simulink library "UserContent_lib"  (Simulink 7.8)
settings: Solver=ode45  SolverMode=SingleTasking  StartTime=0.0  StopTime=10.0  RelTol=1e-3
undefined symbols (not defined in the file): bias, ln, Timestep, u_gain_light, u_gain_moderate, u_gain_severe, v_gain_light, v_gain_moderate, v_gain_severe, w_gain_light, w_gain_moderate, w_gain_severe, WindDir, WindSpd
libraries: simulink x8
(part 2 of 2)

== system UserContent_lib/Input Generator/Winds/Turbulence  Model/Dryden Model/Longitudinal Turbulence/filter parameters/Tm-4511 severe data ==
  note: "Light" and "Moderate" sigmas are ZERO below 1km alt.
      | Table 2-79 does not define them.
  "alt, m" : Inport
  intensity : Inport  Port=2
  "Longitudinal Scale, m TM-4511 Table 2-79" : Lookup  InputValues=[0 10 20 30 40 50 60 70 80 90 100 200 304.8 305 762 769 900 1000 2000 4000 6000 8000 10000 12000 14000 16000]  Table=[21 21 33 43 52 61 68 75 82 89 95 149 196 300 300 533 533 832 902 1040 1040 1040 1230 1800 2820 3400]  SaturateOnIntegerOverflow=on
  "Longitudinal sigma, m/s light TM-4511 Table 2-79" : Lookup  InputValues="[10 20 30 40 50 60 70 80 90 100 200 304.8 305 400  762 769 1000 2000 4000 6000 8000 10000 12000 14000 16000]"  Table="[0   0   0   0   0   0   0   0   0    0    0    0   0   0   0   0   .17  .17  .2   .21   .22   .22   .25   .26   .24   ]"  SaturateOnIntegerOverflow=on
  "Longitudinal sigma, m/s moderate TM-4511 Table 2-79" : Lookup  InputValues="[10 20 30 40 50 60 70 80 90 100 200 304.8 305 400  762 769 1000 2000 4000 6000 8000 10000 12000 14000 16000]"  Table="[0   0  0    0    0   0  0  0   0   0     0    0      0     0      0    0  1.65  1.65 2.04 2.13 2.15 2.23 2.47 2.62 2.44]"  SaturateOnIntegerOverflow=on
  "Longitudinal sigma, m/s severe TM-4511 Table 2-79" : Lookup  InputValues="[10 20 30 40 50 60 70 80 90 100 200 304.8 305 400  762 769 1000 2000 4000 6000 8000 10000 12000 14000 16000]"  Table=[2.31 2.58 2.75 2.88 2.98 3.07 3.15 3.22 3.28 3.33 3.72 3.95 4.37 4.39 4.39 5.7 5.7 5.8 6.24 7.16 7.59 7.72 7.89 6.93 5]  SaturateOnIntegerOverflow=on
  Multiport Switch : MultiPortSwitch  zeroidx=off  SaturateOnIntegerOverflow=on  InputSameDT=on
  "sigma, m/s" : Outport
  "scale length, m" : Outport  Port=2
  wires:
  intensity/1 -> Multiport Switch/1
  "Longitudinal sigma, m/s light TM-4511 Table 2-79"/1 -> Multiport Switch/2
  "Longitudinal sigma, m/s moderate TM-4511 Table 2-79"/1 -> Multiport Switch/3
  "Longitudinal sigma, m/s severe TM-4511 Table 2-79"/1 -> Multiport Switch/4
  Multiport Switch/1 -> "sigma, m/s"/1
  "Longitudinal Scale, m TM-4511 Table 2-79"/1 -> "scale length, m"/1
  "alt, m"/1 -> "Longitudinal sigma, m/s light TM-4511 Table 2-79"/1, "Longitudinal sigma, m/s moderate TM-4511 Table 2-79"/1, "Longitudinal Scale, m TM-4511 Table 2-79"/1, "Longitudinal sigma, m/s severe TM-4511 Table 2-79"/1

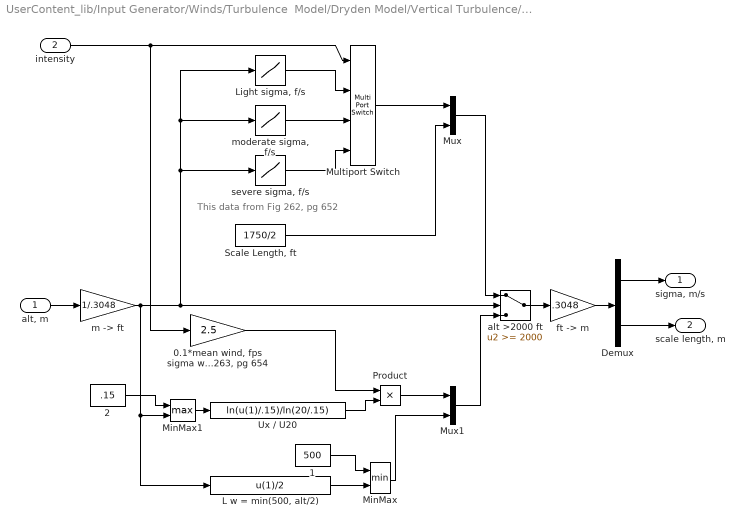
== system UserContent_lib/Input Generator/Winds/Turbulence  Model/Dryden Model/Vertical Turbulence/SubSystem/MIL-STD-1797A APPENDIX A  ==
  note: This data from Fig 262, pg 652
  "alt, m" : Inport
  intensity : Inport  Port=2
  "0.1*mean wind, fps sigma w = to 2.5f/s * intensity Fig 263, pg 654" : Gain  Gain=2.5  SaturateOnIntegerOverflow=on  OutDataTypeStr=Inherit: Same as input  ParamDataTypeStr=Inherit: Same as input
  1 : Constant  Value=500
  2 : Constant  Value=.15
  Demux : Demux  Outputs=2
  "L w = min(500, alt/2)" : Fcn  Expr=u(1)/2
  "Light sigma, f/s" : Lookup  InputValues=[2000 9000 18000 100000]  Table=[5 5 3 3]  SaturateOnIntegerOverflow=on
  MinMax : MinMax  Inputs=2  SaturateOnIntegerOverflow=on  InputSameDT=on
  MinMax1 : MinMax  Function=max  Inputs=2  SaturateOnIntegerOverflow=on  InputSameDT=on
  Multiport Switch : MultiPortSwitch  zeroidx=off  SaturateOnIntegerOverflow=on  InputSameDT=on
  Mux : Mux  Inputs=2
  Mux1 : Mux  Inputs=2
  Product : Product  SaturateOnIntegerOverflow=on  InputSameDT=on  OutDataTypeStr=Inherit: Same as first input
  "Scale Length, ft" : Constant  Value=1750/2
  Ux / U20 : Fcn  Expr=ln(u(1)/.15)/ln(20/.15)
  alt >2000 ft : Switch  Threshold=2000  SaturateOnIntegerOverflow=on  InputSameDT=on
  "ft -> m" : Gain  Gain=.3048  SaturateOnIntegerOverflow=on  OutDataTypeStr=Inherit: Same as input  ParamDataTypeStr=Inherit: Same as input
  "m -> ft" : Gain  Gain=1/.3048  SaturateOnIntegerOverflow=on  OutDataTypeStr=Inherit: Same as input  ParamDataTypeStr=Inherit: Same as input
  "moderate sigma, f/s" : Lookup  InputValues=[2000 12000 44000 100000]  Table=[10 10 3 3]  SaturateOnIntegerOverflow=on
  "severe sigma, f/s" : Lookup  InputValues=[2000 5000 22000 80000 100000]  Table=[15.5 21.5 21.5 3 3]  SaturateOnIntegerOverflow=on
  "sigma, m/s" : Outport
  "scale length, m" : Outport  Port=2
  wires:
  MinMax/1 -> Mux1/2
  Product/1 -> Mux1/1
  "0.1*mean wind, fps sigma w = to 2.5f/s * intensity Fig 263, pg 654"/1 -> Product/1
  Ux / U20/1 -> Product/2
  MinMax1/1 -> Ux / U20/1
  2/1 -> MinMax1/1
  "L w = min(500, alt/2)"/1 -> MinMax/2
  1/1 -> MinMax/1
  "ft -> m"/1 -> Demux/1
  alt >2000 ft/1 -> "ft -> m"/1
  Demux/1 -> "sigma, m/s"/1
  Demux/2 -> "scale length, m"/1
  Mux1/1 -> alt >2000 ft/3
  "m -> ft"/1 -> MinMax1/2, "L w = min(500, alt/2)"/1, "moderate sigma, f/s"/1, "Light sigma, f/s"/1, "severe sigma, f/s"/1, alt >2000 ft/2
  "Scale Length, ft"/1 -> Mux/2
  intensity/1 -> "0.1*mean wind, fps sigma w = to 2.5f/s * intensity Fig 263, pg 654"/1, Multiport Switch/1
  Mux/1 -> alt >2000 ft/1
  Multiport Switch/1 -> Mux/1
  "alt, m"/1 -> "m -> ft"/1
  "severe sigma, f/s"/1 -> Multiport Switch/4
  "moderate sigma, f/s"/1 -> Multiport Switch/3
  "Light sigma, f/s"/1 -> Multiport Switch/2

== system UserContent_lib/Input Generator/Winds/Turbulence  Model/Dryden Model/Vertical Turbulence/SubSystem/Tm-4511 severe data ==
  note: "Light" and "Moderate" sigmas are ZERO below 1km alt.
      | Table 2-79 does not define them.
  "alt, m" : Inport
  intensity : Inport  Port=2
  Multiport Switch : MultiPortSwitch  zeroidx=off  SaturateOnIntegerOverflow=on  InputSameDT=on
  "Vertical sigma, m/s light TM-4511 Table 2-79" : Lookup  InputValues="[10 20 30 40 50 60 70 80 90 100 200 304.8 305 400  762 769 1000 2000 4000 6000 8000 10000 12000 14000 16000]"  Table="[0   0   0   0   0   0   0   0   0    0    0    0   0   0   0   0   .14  .14  .17   .17   .17   .17   .18   .19   .21   ]"  SaturateOnIntegerOverflow=on
  "Vertical sigma, m/s moderate TM-4511 Table 2-79" : Lookup  InputValues="[10 20 30 40 50 60 70 80 90 100 200 304.8 305 400  762 769 1000 2000 4000 6000 8000 10000 12000 14000 16000]"  Table="[0   0  0    0    0   0  0  0   0   0     0    0      0     0      0    0  1.36  1.43 1.68 1.69 1.695 1.73 1.79 1.91 2.1]"  SaturateOnIntegerOverflow=on
  "Vertical  Scale, m TM-4511 Table 2-79" : Lookup  InputValues=[0 10 20 30 40 50 60 70 80 90 100 200 304.8 305 762 769 900 1000 2000 4000 6000 8000 10000 12000 14000 16000]  Table=[ 5 5 11 17 23 29 35 41 47 53 59 123 192 300 300 533 533 624 831 972 1010 980 1100 1540 2120 2600]  SaturateOnIntegerOverflow=on
  "Vertical  sigma, m/s severe TM-4511 Table 2-79" : Lookup  InputValues=[10 20 30 40 50 60 70 80 90 100 200 304.8 305 762 769 900 1000 2000 4000 6000 8000 10000 12000 14000 16000]  Table=[1.15 1.46 1.71 1.89 2.05 2.19 2.32 2.43 2.54 2.64 3.38 3.95 4.39 4.39 5.7 5.7 4.67 4.75 5.13 5.69 5.98 6 5.71 5.05 4.31]  SaturateOnIntegerOverflow=on
  "sigma, m/s" : Outport
  "scale length, m" : Outport  Port=2
  wires:
  "Vertical  sigma, m/s severe TM-4511 Table 2-79"/1 -> Multiport Switch/4
  intensity/1 -> Multiport Switch/1
  "Vertical sigma, m/s light TM-4511 Table 2-79"/1 -> Multiport Switch/2
  "Vertical sigma, m/s moderate TM-4511 Table 2-79"/1 -> Multiport Switch/3
  Multiport Switch/1 -> "sigma, m/s"/1
  "Vertical  Scale, m TM-4511 Table 2-79"/1 -> "scale length, m"/1
  "alt, m"/1 -> "Vertical sigma, m/s light TM-4511 Table 2-79"/1, "Vertical sigma, m/s moderate TM-4511 Table 2-79"/1, "Vertical  sigma, m/s severe TM-4511 Table 2-79"/1, "Vertical  Scale, m TM-4511 Table 2-79"/1
